simulink subsystem "hexa_aero_forces_moments"  (R2024a)
settings: Solver=VariableStepAuto  StartTime=0.0  StopTime=10.0  RelTol=1e-3
values from neighbouring files (symbols this model uses):
  Cd = 0.25    [F550_data.m]
  Cmd = [0.0035 0.0039 0.0034]    [F550_data.m]
  dzcg = 0.12    [F550_data.m]
settings Model: Creator=user  LastModifiedBy=user

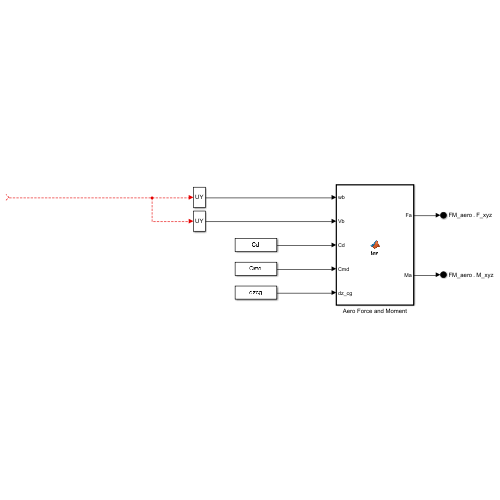
[thumbnail: Simulink's stored preview of the top-level diagram]
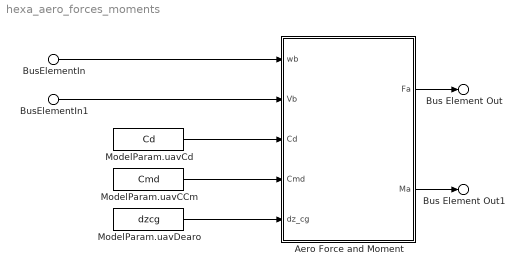
== system hexa_aero_forces_moments ==
  BusElementIn : Inport  PortName=States  Element=PQR
  BusElementIn1 : Inport  PortName=States  Element=UVWb
  Aero Force and Moment : MATLAB Function  TreatAsAtomicUnit=on
  ModelParam.uavCCm : Constant  Value=Cmd
  ModelParam.uavCd : Constant  Value=Cd
  ModelParam.uavDearo : Constant  Value=dzcg
  Bus Element Out : Outport  PortName=FM_aero  Element=F_xyz
  Bus Element Out1 : Outport  PortName=FM_aero  Element=M_xyz
  wires:
  Aero Force and Moment/2(Ma) -> Bus Element Out1/1
  ModelParam.uavCCm/1 -> Aero Force and Moment/4(Cmd)
  ModelParam.uavCd/1 -> Aero Force and Moment/3(Cd)
  BusElementIn/1 -> Aero Force and Moment/1(wb)
  ModelParam.uavDearo/1 -> Aero Force and Moment/5(dz_cg)
  Aero Force and Moment/1(Fa) -> Bus Element Out/1
  BusElementIn1/1 -> Aero Force and Moment/2(Vb)

== matlab function hexa_aero_forces_moments/Aero Force and Moment ==
  data: Fa output; Ma output; wb input; Vb input; Cd input; Cmd input; dz_cg input
function [Fa,Ma] = fcn(wb,Vb,Cd,Cmd,dz_cg)

 Fa = -Cd*Vb.*abs(Vb);         % Careful for the definition of Cd

 Md = -Cmd.*wb.*abs(wb);       % aerodynamic damping moment
  
 Mfd= [Fa(2)*dz_cg
      -Fa(1)*dz_cg
       0];

 Ma = Mfd + Md;
 %Ma = Md; % Ignore Damping moment
end
